simulink model "SetPosition_2016"  (Simulink 8.8)
settings: Solver=FixedStepAuto  StartTime=0.0  StopTime=15.0  FixedStep=Config.Ts  RelTol=1e-3
StopFcn:
  | save(['Data/Unmergeddata/',configjoint,num2str(A),'A',num2str(f),'F',datestr(now,'dd-mm-yy HH:MM:SS'),'.mat']);
undefined symbols (not defined in the file): A, Config, f
libraries: WBToolboxLibrary x15
settings Model: SuppressorTable=22 serialization::archive 11 0 6 0 0 0 11 0  Creator=vaggarwal  LastModifiedBy=vaggarwal
settings DataIOCC: LimitDataPoints=off  SaveFormat=Dataset  SignalLoggingSaveFormat=Dataset
settings OptimizationCC: LifeSpan=auto
settings DebuggingCC: UnderspecifiedInitializationDetection=Simplified  MergeDetectMultiDrivingBlocksExec=error  InheritedTsInSrcMsg=none  FcnCallInpInsideContextMsg=error  StateNameClashWarn=none  SFUnexpectedBacktrackingDiag=error  SFNoUnconditionalDefaultTransitionDiag=error  SFExecutionAtInitializationDiag=warning
settings HardwareCC: ProdBitPerPointer=64  ProdBitPerSizeT=64  ProdBitPerPtrDiffT=64  ProdLargestAtomicFloat=Float  ProdIntDivRoundTo=Zero  ProdEndianess=LittleEndian  ProdWordSize=64  ProdHWDeviceType=Intel->x86-64 (Windows64)
settings ModelReferenceCC: PropagateSignalLabelsOutOfModel=on
settings GRTTargetCC: TargetLangStandard=C99 (ISO)  GeneratePreprocessorConditionals=Use local settings  CombineOutputUpdateFcns=on  GRTInterface=off
settings ConfigComp: CovMetricSettings=dwe  CovHtmlReporting=off  CovSaveCumulativeToWorkspaceVar=off  CovSaveSingleToWorkspaceVar=off  CovExternalEMLEnable=on

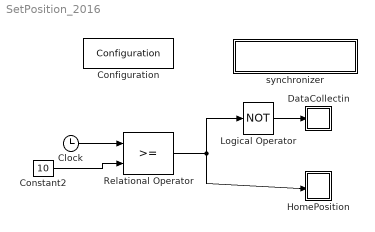
== system SetPosition_2016 ==
  Clock : Clock
  Configuration : WBToolboxLibrary/Utilities/Configuration  ConfigSource=Mask  ConfigObject='WBTConfigRobot'  RobotName='icub'  UrdfFile='model.urdf'  ControlledJoints={configjoint}  ControlBoardsNames={'left_leg','right_leg'}  LocalName='WBT'  GravityVector=[0,0,-9.81]
  Constant2 : Constant  Value=10
  DataCollectin : Subsystem  TreatAsAtomicUnit=on
  HomePosition : Subsystem  TreatAsAtomicUnit=on
  Logical Operator : Logic  Operator=NOT  AllPortsSameDT=off  OutDataTypeStr=boolean
  Relational Operator : RelationalOperator  OutDataTypeStr=boolean  RndMeth=Simplest
  synchronizer : Subsystem
      mask Display: disp('SYNCHRONIZER')
  wires:
  Clock/1 -> Relational Operator/1
  Constant2/1 -> Relational Operator/2
  Relational Operator/1 -> HomePosition/Enable, Logical Operator/1
  Logical Operator/1 -> DataCollectin/Enable

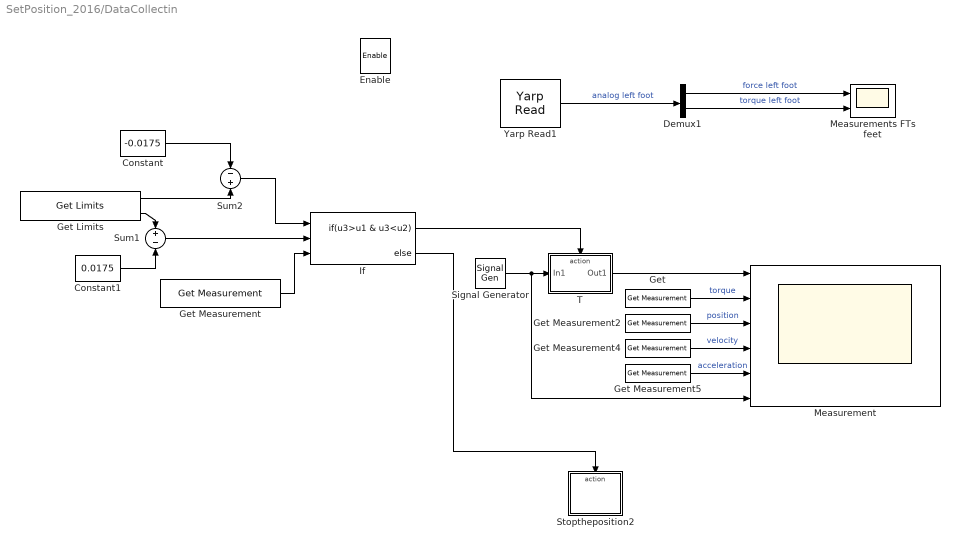
== system SetPosition_2016/DataCollectin ==
  Enable : EnablePort
  Constant : Constant  Value=-0.0175
  Constant1 : Constant  Value=0.0175
  Demux1 : Demux  Outputs=2
  "Get " : WBToolboxLibrary/wholeBodyStates/Get Measurement  measuredType=Joints Torque
  Get Limits : WBToolboxLibrary/wholeBodyStates/Get Limits  limitsSource=ControlBoard  limitsType=Position
  Get Measurement : WBToolboxLibrary/wholeBodyStates/Get Measurement  measuredType=Joints Position
  Get Measurement2 : WBToolboxLibrary/wholeBodyStates/Get Measurement  measuredType=Joints Position
  Get Measurement4 : WBToolboxLibrary/wholeBodyStates/Get Measurement  measuredType=Joints Velocity
  Get Measurement5 : WBToolboxLibrary/wholeBodyStates/Get Measurement  measuredType=Joints Acceleration
  If : If  NumInputs=3  IfExpression=u3>u1 & u3<u2
  "Measurement " : Scope  NumInputPorts=6
  Measurements FTs feet : Scope  NumInputPorts=2
  Signal Generator : SignalGenerator  WaveForm=square  Amplitude=A  Frequency=f
  Stoptheposition2 : Subsystem
  Sum1 : Sum  Inputs=+|-
  Sum2 : Sum  Inputs=-|+
  T : Subsystem
  Yarp Read1 : WBToolboxLibrary/Utilities/Yarp Read  portName='/icub/left_foot/analog:o'  signalSize=6  timeout=0.5  blocking=off  timestamp=off  autoconnect=on  errorOnConnection=off
  wires:
  If/1 -> T/Action
  Signal Generator/1 -> T/1(In1), "Measurement "/6
  Get Measurement5/1 -> "Measurement "/5  "acceleration"
  Get Measurement2/1 -> "Measurement "/3  "position"
  "Get "/1 -> "Measurement "/2  "torque"
  Get Measurement4/1 -> "Measurement "/4  "velocity"
  T/1(Out1) -> "Measurement "/1
  Get Measurement/1 -> If/3
  Get Limits/1 -> Sum2/2
  Constant/1 -> Sum2/1
  Get Limits/2 -> Sum1/1
  Constant1/1 -> Sum1/2
  Sum1/1 -> If/2
  Sum2/1 -> If/1
  If/2 -> Stoptheposition2/Action
  Demux1/1 -> Measurements FTs feet/1  "force left foot"
  Demux1/2 -> Measurements FTs feet/2  "torque left foot"
  Yarp Read1/1 -> Demux1/1  "analog left foot"

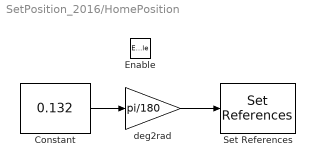
== system SetPosition_2016/HomePosition ==
  Enable : EnablePort
  Constant : Constant  Value=0.132
  Set References : WBToolboxLibrary/wholeBodyActuators/Set References  controlType=Position  refSpeed=50
  deg2rad : Gain  Gain=pi/180
  wires:
  Constant/1 -> deg2rad/1
  deg2rad/1 -> Set References/1

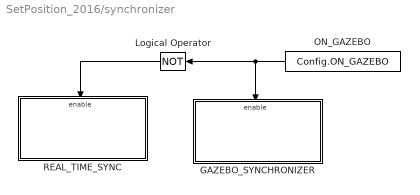
== system SetPosition_2016/synchronizer ==
  GAZEBO_SYNCHRONIZER : Subsystem
  Logical Operator : Logic  Operator=NOT  AllPortsSameDT=off  OutDataTypeStr=boolean
  "ON_GAZEBO " : Constant  Value=Config.ON_GAZEBO
  REAL_TIME_SYNC : Subsystem
  wires:
  Logical Operator/1 -> REAL_TIME_SYNC/Enable
  "ON_GAZEBO "/1 -> GAZEBO_SYNCHRONIZER/Enable, Logical Operator/1

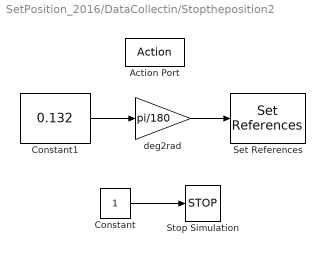
== system SetPosition_2016/DataCollectin/Stoptheposition2 ==
  Action Port : ActionPort  ActionType=else
  Constant : Constant
  Constant1 : Constant  Value=0.132
  Set References : WBToolboxLibrary/wholeBodyActuators/Set References  controlType=Position  refSpeed=10
  Stop Simulation : Stop
  deg2rad : Gain  Gain=pi/180
  wires:
  Constant/1 -> Stop Simulation/1
  Constant1/1 -> deg2rad/1
  deg2rad/1 -> Set References/1

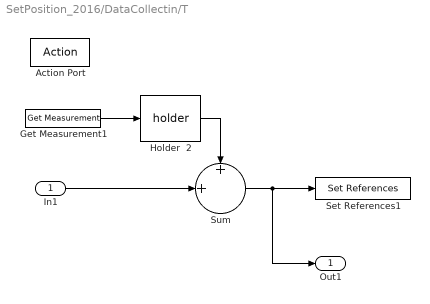
== system SetPosition_2016/DataCollectin/T ==
  In1 : Inport
  Action Port : ActionPort  ActionType=then
  Get Measurement1 : WBToolboxLibrary/wholeBodyStates/Get Measurement  measuredType=Joints Torque
  Holder  2 : WBToolboxLibrary/Utilities/holder 
  Set References1 : WBToolboxLibrary/wholeBodyActuators/Set References  controlType=Position  refSpeed=40
  Sum : Sum  Inputs=+|+||
  Out1 : Outport
  wires:
  Sum/1 -> Out1/1, Set References1/1
  Get Measurement1/1 -> Holder  2/1
  Holder  2/1 -> Sum/1
  In1/1 -> Sum/2

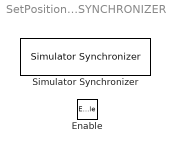
== system SetPosition_2016/synchronizer/GAZEBO_SYNCHRONIZER ==
  Enable : EnablePort
  Simulator Synchronizer : WBToolboxLibrary/Utilities/Simulator Synchronizer  period=Config.Ts  serverPortName='/clock/rpc'  clientPortName='/WBT_synchronizer/rpc:o'

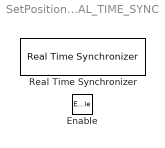
== system SetPosition_2016/synchronizer/REAL_TIME_SYNC ==
  Enable : EnablePort
  Real Time Synchronizer : WBToolboxLibrary/Utilities/Real Time Synchronizer  period=Config.Ts
